simulink model "nogimbangle_cilinder"  (R2024b)
settings: Solver=VariableStepAuto  StartTime=0.0  StopTime=100  RelTol=1e-3
PreLoadFcn:
  | A = 0.09*pi; % Frontal area
  | C_D = 0.6; % Drag coefficient
  | p = 1.225; % Air density
values from neighbouring files (symbols this model uses):
  m_p = 70    [rocketsim.m]    (also in simulinkrocket.m)
  m_s = 30    [rocketsim.m]    (also in simulinkrocket.m)
  T = 1000    [rocketsim.m]    (also in simulinkrocket.m)
  t_b = 15    [rocketsim.m]    (also in simulinkrocket.m)
libraries: simulink x1
settings Model: Creator=User  LastModifiedBy=User
settings DebuggingCC: AlgebraicLoopMsg=none

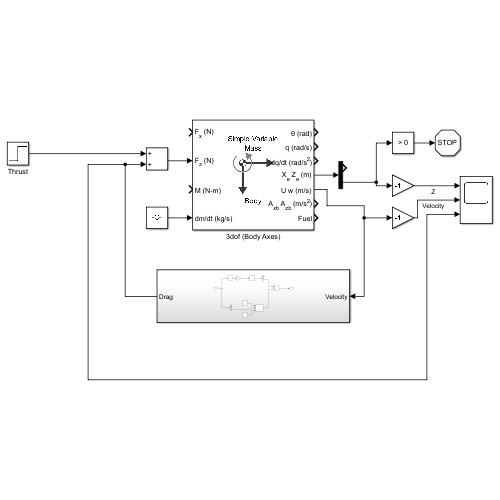
[thumbnail: Simulink's stored preview of the top-level diagram]
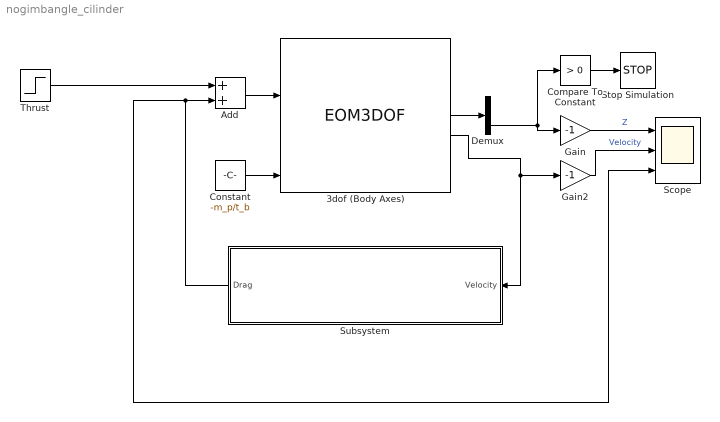
== system nogimbangle_cilinder ==
  3dof (Body Axes) : EOM3DOF  mtype=Simple Variable  v_ini=0  mass=m_s+m_p  mass_e=m_s  mass_f=m_s+m_p  Iyy=0.048  Iyy_e=I_s  Iyy_f=I_p
  Add : Sum
  Compare To Constant : simulink/Logic and Bit Operations/Compare To Constant  relop=>  const=0  OutDataTypeStr=boolean
  Constant : Constant  Value=-m_p/t_b
  Demux : Demux  Outputs=2
  Gain : Gain  Gain=-1
  Gain2 : Gain  Gain=-1
  Scope : Scope  NumInputPorts=3
  Stop Simulation : Stop
  Subsystem : Subsystem
  Thrust : Step  Time=t_b  Before=-T  After=0  SampleTime=0
  wires:
  Thrust/1 -> Add/1
  3dof (Body Axes)/4 -> Demux/1
  Compare To Constant/1 -> Stop Simulation/1
  Gain/1 -> Scope/1  "Z"
  Demux/2 -> Gain/1, Compare To Constant/1
  3dof (Body Axes)/5 -> Gain2/1, Subsystem/1(Velocity)
  Constant/1 -> 3dof (Body Axes)/4
  Add/1 -> 3dof (Body Axes)/2
  Gain2/1 -> Scope/2  "Velocity"
  Subsystem/1(Drag) -> Add/2, Scope/3

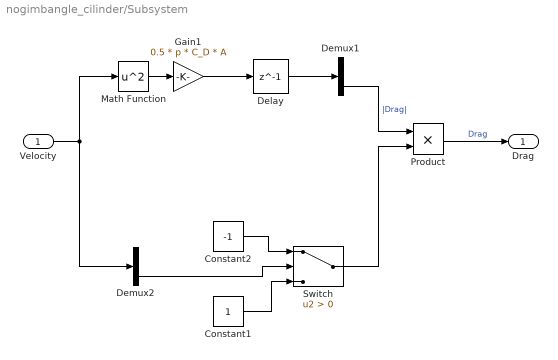
== system nogimbangle_cilinder/Subsystem ==
  Velocity : Inport
  Constant1 : Constant
  Constant2 : Constant  Value=-1
  Delay : Delay  DelayLength=1  SampleTime=0.001
  Demux1 : Demux  Outputs=2
  Demux2 : Demux  Outputs=2
  Gain1 : Gain  Gain=0.5 * p * C_D * A
  Math Function : Math  Operator=square
  Product : Product
  Switch : Switch  Criteria=u2 > Threshold  SaturateOnIntegerOverflow=off  InputSameDT=off
  Drag : Outport
  wires:
  Math Function/1 -> Gain1/1
  Demux1/2 -> Product/1  "|Drag|"
  Gain1/1 -> Delay/1
  Demux2/2 -> Switch/2
  Velocity/1 -> Math Function/1, Demux2/1
  Constant2/1 -> Switch/1
  Delay/1 -> Demux1/1
  Switch/1 -> Product/2
  Constant1/1 -> Switch/3
  Product/1 -> Drag/1  "Drag"
